simulink model "matrix_for_each_wrapper"  (R2025b)
settings: Solver=FixedStepDiscrete  StartTime=0.0  StopTime=10.0  RelTol=1e-3
settings Model: Creator=aherrman  LastModifiedBy=aherrman
settings OptimizationCC: DefaultParameterBehavior=Inlined

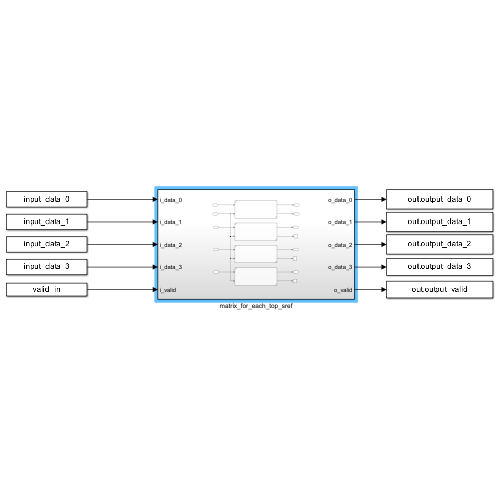
[thumbnail: Simulink's stored preview of the top-level diagram]
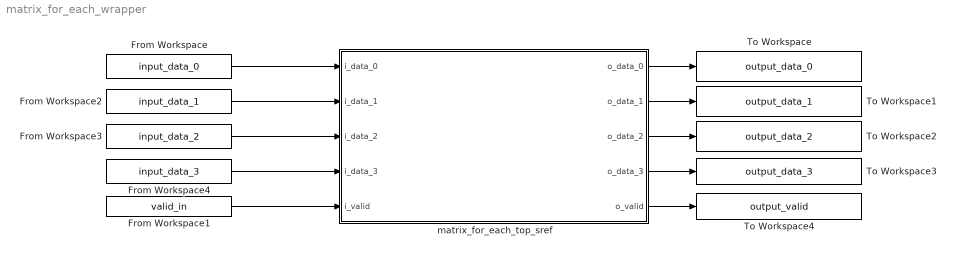
== system matrix_for_each_wrapper ==
  From Workspace : FromWorkspace  VariableName=input_data_0  SampleTime=1  Interpolate=off  ZeroCross=off  OutputAfterFinalValue=Setting to zero
  From Workspace1 : FromWorkspace  VariableName=valid_in  SampleTime=1  Interpolate=off  ZeroCross=off  OutputAfterFinalValue=Setting to zero
  From Workspace2 : FromWorkspace  VariableName=input_data_1  SampleTime=1  Interpolate=off  ZeroCross=off  OutputAfterFinalValue=Setting to zero
  From Workspace3 : FromWorkspace  VariableName=input_data_2  SampleTime=1  Interpolate=off  ZeroCross=off  OutputAfterFinalValue=Setting to zero
  From Workspace4 : FromWorkspace  VariableName=input_data_3  SampleTime=1  Interpolate=off  ZeroCross=off  OutputAfterFinalValue=Setting to zero
  To Workspace : ToWorkspace  VariableName=output_data_0  SaveFormat=Timeseries  SampleTime=-1
  To Workspace1 : ToWorkspace  VariableName=output_data_1  SaveFormat=Timeseries  SampleTime=-1
  To Workspace2 : ToWorkspace  VariableName=output_data_2  SaveFormat=Timeseries  SampleTime=-1
  To Workspace3 : ToWorkspace  VariableName=output_data_3  SaveFormat=Timeseries  SampleTime=-1
  To Workspace4 : ToWorkspace  VariableName=output_valid  SaveFormat=Timeseries  SampleTime=-1
  matrix_for_each_top_sref : Subsystem
  wires:
  From Workspace/1 -> matrix_for_each_top_sref/1(i_data_0)
  From Workspace1/1 -> matrix_for_each_top_sref/5(i_valid)
  matrix_for_each_top_sref/1(o_data_0) -> To Workspace/1
  matrix_for_each_top_sref/4(o_data_3) -> To Workspace3/1
  matrix_for_each_top_sref/3(o_data_2) -> To Workspace2/1
  matrix_for_each_top_sref/2(o_data_1) -> To Workspace1/1
  From Workspace2/1 -> matrix_for_each_top_sref/2(i_data_1)
  From Workspace3/1 -> matrix_for_each_top_sref/3(i_data_2)
  From Workspace4/1 -> matrix_for_each_top_sref/4(i_data_3)
  matrix_for_each_top_sref/5(o_valid) -> To Workspace4/1

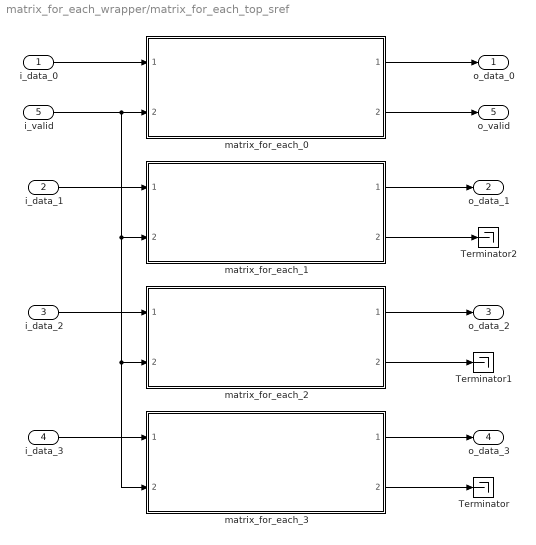
== system matrix_for_each_wrapper/matrix_for_each_top_sref ==
  i_data_0 : Inport
  i_data_1 : Inport  Port=2
  i_data_2 : Inport  Port=3
  i_data_3 : Inport  Port=4
  i_valid : Inport  Port=5
  Terminator : Terminator
  Terminator1 : Terminator
  Terminator2 : Terminator
  matrix_for_each_{0..3} (4 alike) : Subsystem  ReferencedSubsystem=matrix_for_each_sref
  o_data_0 : Outport
  o_data_1 : Outport  Port=2
  o_data_2 : Outport  Port=3
  o_data_3 : Outport  Port=4
  o_valid : Outport  Port=5
  wires:
  i_data_1/1 -> matrix_for_each_1/1
  matrix_for_each_0/1 -> o_data_0/1
  i_data_0/1 -> matrix_for_each_0/1
  i_data_2/1 -> matrix_for_each_2/1
  matrix_for_each_1/1 -> o_data_1/1
  i_data_3/1 -> matrix_for_each_3/1
  matrix_for_each_2/1 -> o_data_2/1
  i_valid/1 -> matrix_for_each_0/2, matrix_for_each_3/2, matrix_for_each_2/2, matrix_for_each_1/2
  matrix_for_each_3/1 -> o_data_3/1
  matrix_for_each_3/2 -> Terminator/1
  matrix_for_each_2/2 -> Terminator1/1
  matrix_for_each_1/2 -> Terminator2/1
  matrix_for_each_0/2 -> o_valid/1
